simulink model "shareefprojectwork"  (Simulink 6.6)
settings: Solver=ode45  StartTime=0.0  StopTime=0.1  RelTol=1e-3
libraries: powerlib x12
settings Model: Creator=Y9EE1238  LastModifiedBy=Y9EE1238

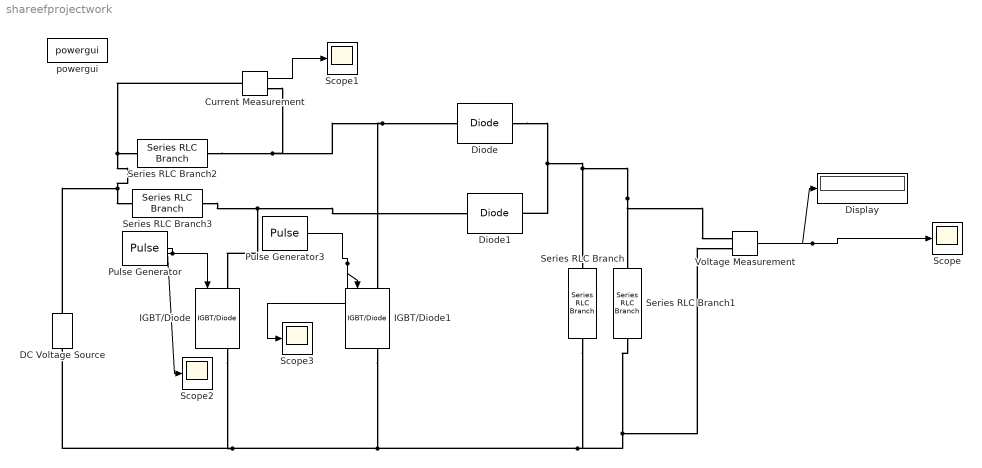
== system shareefprojectwork ==
  Current Measurement : powerlib/Measurements/Current Measurement  DialogController=POWERSYS.PowerSysDialog  SystemSampleTime=-1  PhasorSimulation=off  OutputType=Complex  PSBequivalent=0
  DC Voltage Source : powerlib/Electrical Sources/DC Voltage Source  Orientation=up  DialogController=POWERSYS.PowerSysDialog  SystemSampleTime=-1  Amplitude=20  Measurements=None
  Diode : powerlib/Power Electronics/Diode  DialogController=POWERSYS.PowerSysDialog  SystemSampleTime=-1  Ron=0.001  Lon=0  Vf=0.8  IC=0  Rs=500  Cs=250e-9  Measurements=off
  Diode1 : powerlib/Power Electronics/Diode  DialogController=POWERSYS.PowerSysDialog  SystemSampleTime=-1  Ron=0.001  Lon=0  Vf=0.8  IC=0  Rs=500  Cs=250e-9  Measurements=off
  Display : Display
  IGBT/Diode : powerlib/Power Electronics/IGBT//Diode  Orientation=down  DialogController=POWERSYS.PowerSysDialog  SystemSampleTime=-1  Ron=1e-3  Rs=1e5  Cs=inf  Measurements=on
  IGBT/Diode1 : powerlib/Power Electronics/IGBT//Diode  Orientation=down  DialogController=POWERSYS.PowerSysDialog  SystemSampleTime=-1  Ron=1e-3  Rs=1e5  Cs=inf  Measurements=on
  Pulse Generator : DiscretePulseGenerator  PulseType=Time based  Period=0.0005  PulseWidth=50
  Pulse Generator3 : DiscretePulseGenerator  PulseType=Time based  Period=0.0005  PulseWidth=50  PhaseDelay=0.00025
  Scope{,1..3} (4 alike) : Scope
      Scope settings: TimeRange=0.1  YMin=41  YMax=42.5  SaveName=miskin
      Scope1 settings: YMin=5  YMax=27.5
      Scope2 settings: YMin=0  YMax=0.01  SaveName=ScopeData2
      Scope3 settings: YMin=0  YMax=0.01  SaveName=ScopeData3
  Series RLC Branch : powerlib/Elements/Series RLC Branch  Orientation=down  DialogController=POWERSYS.PowerSysDialog  PhysicalDomain=powersysdomain  SubClassName=unknown  LeftPortType=p1  RightPortType=p1  LConnTagsString=__new0  RConnTagsString=__new0  BranchType=C  Resistance=1  Inductance=1e-3  SetiL0=off  InitialCurrent=0  Capacitance=750e-6  Setx0=off  InitialVoltage=39  Measurements=None
  Series RLC Branch1 : powerlib/Elements/Series RLC Branch  Orientation=down  DialogController=POWERSYS.PowerSysDialog  PhysicalDomain=powersysdomain  SubClassName=unknown  LeftPortType=p1  RightPortType=p1  LConnTagsString=__new0  RConnTagsString=__new0  BranchType=R  Resistance=16  Inductance=1e-3  SetiL0=off  InitialCurrent=0  Capacitance=1e-6  Setx0=off  InitialVoltage=0  Measurements=None
  Series RLC Branch2 : powerlib/Elements/Series RLC Branch  DialogController=POWERSYS.PowerSysDialog  PhysicalDomain=powersysdomain  SubClassName=unknown  LeftPortType=p1  RightPortType=p1  LConnTagsString=__new0  RConnTagsString=__new0  BranchType=L  Resistance=1  Inductance=6.8e-3  SetiL0=off  InitialCurrent=20  Capacitance=1e-6  Setx0=off  InitialVoltage=0  Measurements=None
  Series RLC Branch3 : powerlib/Elements/Series RLC Branch  DialogController=POWERSYS.PowerSysDialog  PhysicalDomain=powersysdomain  SubClassName=unknown  LeftPortType=p1  RightPortType=p1  LConnTagsString=__new0  RConnTagsString=__new0  BranchType=L  Resistance=1  Inductance=6.8e-3  SetiL0=off  InitialCurrent=20  Capacitance=1e-6  Setx0=off  InitialVoltage=0  Measurements=None
  Voltage Measurement : powerlib/Measurements/Voltage Measurement  DialogController=POWERSYS.PowerSysDialog  SystemSampleTime=-1  PhasorSimulation=off  OutputType=Complex  PSBequivalent=0
  powergui : powerlib/powergui  SystemSampleTime=-1  SimulationMode=Discrete  SampleTime=50e-9  echomessages=on  RestoreLinks=warning  x0status=blocks  Frange=[0:2:500]  Ylog=off  Xlog=on  ShowGrid=off  save=off  variable=ZData  structure=miskin  ZoomFFT=off  StartTime=0.0  cycles=1  DisplayStyle=4  fundamental=60  FreqAxis=off  MaxFrequency=1000  frequencyindice=0  frequencyindicesteady=1  RmsSteady=1  display=off  Ts=0  frequency=60  methode=off  HookPort=off  Interpol=off
  wires:
  Pulse Generator/1 -> IGBT/Diode/1, Scope2/1
  Current Measurement/1 -> Scope1/1
  Voltage Measurement/1 -> Scope/1, Display/1
  Pulse Generator3/1 -> IGBT/Diode1/1, Scope3/1
  connections:
  Series RLC Branch3/LConn1 -- Current Measurement/LConn1 -- Series RLC Branch2/LConn1 -- DC Voltage Source/RConn1
  Series RLC Branch3/RConn1 -- Diode1/LConn1 -- IGBT/Diode/LConn1
  Series RLC Branch2/RConn1 -- Diode/LConn1 -- IGBT/Diode1/LConn1 -- Current Measurement/RConn1
  Diode/RConn1 -- Diode1/RConn1 -- Series RLC Branch/LConn1 -- Series RLC Branch1/LConn1 -- Voltage Measurement/LConn1
  Series RLC Branch/RConn1 -- Series RLC Branch1/RConn1 -- Voltage Measurement/LConn2 -- DC Voltage Source/LConn1 -- IGBT/Diode/RConn1 -- IGBT/Diode1/RConn1
